simulink subsystem "PID_Control_Subsystem"  (R2023a)
settings: Solver=VariableStepAuto  StartTime=0.0  StopTime=10.0  RelTol=1e-3
values from neighbouring files (symbols this model uses):
  A = [0      1       0           0 ... (first row only)    [MS_PID_Control.m]    (also in PID_Control.m = [0      1       0)
  B = [0 k_m/m1 0 1/m2]'    [MS_PID_Control.m]    (also in PID_Control.m = [0 0 1/L]')
  C = [-k1/m1 -c1/m1   k1/m1       c1/m1 ... (first row only)    [MS_PID_Control.m]    (also in PID_Control.m = [-k/m -c/m k_M/m])
  D = 0    [MS_PID_Control.m]    (also in PID_Control.m)
  E = [0 0 0 c2/m2 ... (first row only)    [MS_PID_Control.m]    (also in PID_Control.m = [0      0)
  Kd = 00070    (= 70)    [MS_PID_Control.m]    (also in PID_Control.m)
  Ki = 13000    [MS_PID_Control.m]    (also in PID_Control.m)
  Kp = 27000    [MS_PID_Control.m]    (also in PID_Control.m)
libraries: slpidlib x1
settings Model: Creator=z'k'x  LastModifiedBy=z'k'x

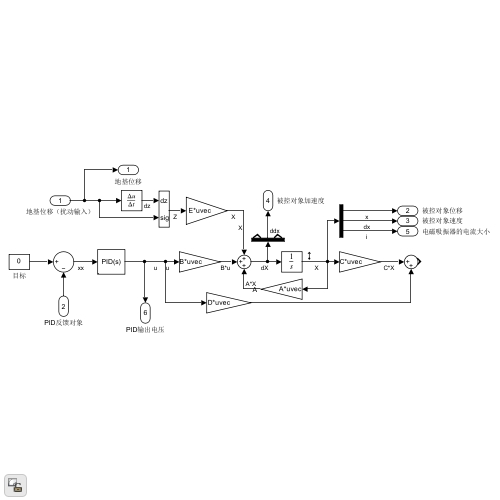
[thumbnail: Simulink's stored preview of the top-level diagram]
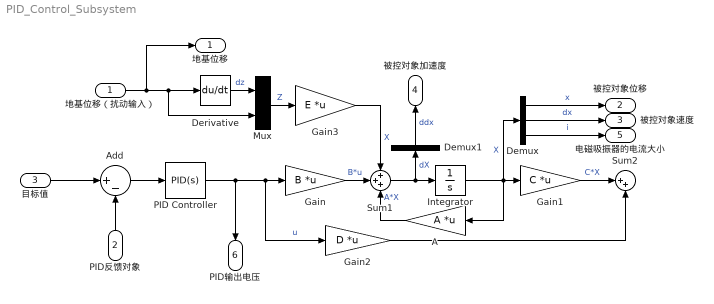
== system PID_Control_Subsystem ==
  地基位移（扰动输入） : Inport
  PID反馈对象 : Inport  Port=2
  目标值 : Inport  Port=3
  A : Gain  Gain=A  Multiplication=Matrix(K*u) (u vector)
  Add : Sum  Inputs=|+-
  Demux : Demux  Outputs=3
  Demux1 : Demux  Outputs=3
  Derivative : Derivative
  Gain : Gain  Gain=B  Multiplication=Matrix(K*u) (u vector)
  Gain1 : Gain  Gain=C  Multiplication=Matrix(K*u) (u vector)
  Gain2 : Gain  Gain=D  Multiplication=Matrix(K*u) (u vector)
  Gain3 : Gain  Gain=E  Multiplication=Matrix(K*u) (u vector)
  Integrator : Integrator
  Mux : Mux  Inputs=2
      settings: DisplayOption=signals
  PID Controller : slpidlib/PID Controller  Controller=PID  Form=Parallel  TimeDomain=Continuous-time  UseExternalTs=off  SampleTime=-1  IntegratorMethod=Forward Euler  FilterMethod=Forward Euler  ControllerParametersSource=internal  P=Kp  I=Ki  UseKiTs=off  D=Kd  N=100  UseFilter=on  TunerSelectOption=Transfer Function Based (PID Tuner App)  InitialConditionSource=internal  InitialConditionForIntegrator=0  InitialConditionForFilter=0  DifferentiatorICPrevScaledInput=0  ExternalReset=none  TrackingMode=off  Kt=1  LimitOutput=off  SatLimitsSource=internal  UpperSaturationLimit=inf  LowerSaturationLimit=-inf  LinearizeAsGain=on  AntiWindupMode=none  Kb=1  LimitIntegrator=off  UpperIntegratorSaturationLimit=inf  LowerIntegratorSaturationLimit=-inf  POutMin=[]  POutMax=[]  IOutMin=[]  IOutMax=[]  DOutMin=[]  DOutMax=[]  NOutMin=[]  NOutMax=[]  SumOutMin=[]  SumOutMax=[]  SaturationOutMin=[]  SaturationOutMax=[]  PParamMin=[]  PParamMax=[]  IParamMin=[]  IParamMax=[]  DParamMin=[]  DParamMax=[]  NParamMin=[]  NParamMax=[]  KbParamMin=[]  KbParamMax=[]  KtParamMin=[]  KtParamMax=[]  KbOutMin=[]  KbOutMax=[]  KtOutMin=[]  KtOutMax=[]  IntegratorOutMin=[]  IntegratorOutMax=[]  FilterOutMin=[]  FilterOutMax=[]  SumI1OutMin=[]  SumI1OutMax=[]  SumI2OutMin=[]  SumI2OutMax=[]  SumI3OutMin=[]  SumI3OutMax=[]  SumI4OutMin=[]  SumI4OutMax=[]  SumDOutMin=[]  SumDOutMax=[]  DifferentiatorOutMin=[]  DifferentiatorOutMax=[]  FilterDiffOutCoefMin=[]  FilterDiffOutCoefMax=[]  ReciprocalOutMin=[]  ReciprocalOutMax=[]  SumDenOutMin=[]  SumDenOutMax=[]  SumNumOutMin=[]  SumNumOutMax=[]  DivideOutMin=[]  DivideOutMax=[]  UdiffTsProdOutMin=[]  UdiffTsProdOutMax=[]  NTsProdOutMin=[]  NTsProdOutMax=[]  UintegralTsProdOutMin=[]  UintegralTsProdOutMax=[]  UngainTsProdOutMin=[]  UngainTsProdOutMax=[]  ClampingZeroOutDataTypeStr=Inherit: Inherit via back propagation  ClampingZeroOutMin=[]  ClampingZeroOutMax=[]  FilterDenConstantOutDataTypeStr=Inherit: Inherit via back propagation  FilterDenConstantOutMin=[]  FilterDenConstantOutMax=[]  PCopyOutDataTypeStr=Inherit: Inherit via back propagation  PCopyOutMin=[]  PCopyOutMax=[]  NCopyOutDataTypeStr=Inherit: Inherit via back propagation  NCopyOutMin=[]  NCopyOutMax=[]  IntegratorContinuousStateAttributes=''  IntegratorStateMustResolveToSignalObject=off  IntegratorRTWStateStorageClass=Auto  FilterContinuousStateAttributes=''  FilterStateMustResolveToSignalObject=off  FilterRTWStateStorageClass=Auto  ParallelPVariant=InternalParameters  IdealPVariant=Disabled  IVariant=InternalParameters  DVariant=InternalParameters  IntegratorVariant=Continuous  SatVariant=Disabled  AWVariant=Passthrough  PCopyVariant=Disabled  TRVariant=Disabled  FdbkBlocksVariant=Forward  IdealPFdbkVariant=Disabled  SatFdbkVariant=Disabled  DerivativeFilterVariant=ContFilter  NVariant=InternalParameters  NCopyVariant=Disabled  FilterICVariant=InternalICsFilter  IntegratorICVariant=InternalICs  ExternalResetVariant=Disabled  TRSumVariant=Passthrough  SumFdbkVariant=Disabled  SumVariant=Sum_PID  TsampFilterVariant=InternalTs  TsampNgainVariant=Passthrough  TsampIntegralVariant=Disabled_SignalSpec  ExternalSaturationOutDataTypeStr=Inherit: Same as second input
  Sum1 : Sum  Inputs=+++
  Sum2 : Sum  Inputs=|++
  地基位移 : Outport
  被控对象位移 : Outport  Port=2
  被控对象速度 : Outport  Port=3
  被控对象加速度 : Outport  Port=4
  电磁吸振器的电流大小 : Outport  Port=5
  PID输出电压 : Outport  Port=6
  wires:
  目标值/1 -> Add/1
  Demux/3 -> 电磁吸振器的电流大小/1  "i"
  Demux/2 -> 被控对象速度/1  "dx"
  Sum1/1 -> Demux1/1, Integrator/1  "dX"
  Integrator/1 -> Demux/1, Gain1/1, A/1  "X"
  地基位移（扰动输入）/1 -> Mux/2, Derivative/1, 地基位移/1
  A/1 -> Sum1/3  "A*X"
  Gain/1 -> Sum1/2  "B*u"
  Gain1/1 -> Sum2/1  "C*X"
  Demux/1 -> 被控对象位移/1  "x"
  PID Controller/1 -> Gain/1, Gain2/1, PID输出电压/1  "u"
  Gain3/1 -> Sum1/1  "X"
  Derivative/1 -> Mux/1  "dz"
  PID反馈对象/1 -> Add/2
  Add/1 -> PID Controller/1
  Mux/1 -> Gain3/1  "Z"
  Gain2/1 -> Sum2/2
  Demux1/2 -> 被控对象加速度/1  "ddx"
